simulink model "DigitalControlTestCase"  (R2017b)
settings: Solver=VariableStepAuto  StartTime=0.0  StopTime=inf  RelTol=1e-3
libraries: DigiConLib x3
settings Model: Creator=alexandersoussan  LastModifiedBy=alexandersoussan

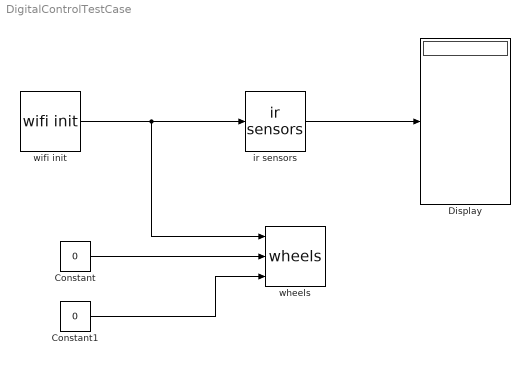
== system DigitalControlTestCase ==
  Constant : Constant  Value=0
  Constant1 : Constant  Value=0
  Display : Display
  ir sensors : DigiConLib/ir sensors
  wheels : DigiConLib/wheels
  wifi init : DigiConLib/wifi init
  wires:
  wifi init/1 -> ir sensors/1, wheels/1
  Constant/1 -> wheels/2
  Constant1/1 -> wheels/3
  ir sensors/1 -> Display/1
